simulink model "OFDM_Rx"  (R2025b)
settings: Solver=FixedStepAuto  StartTime=0.0  StopTime=10  RelTol=1e-3
undefined symbols (not defined in the file): Fs, ip, usb
libraries: commofdm x5, hdlsllib x4, plutoradiolib x2, commseqgen3 x2, commchan3 x1, commutil2 x1, commdigbbndpm3 x1, commrandsrc3 x1
settings Model: Creator=joann  LastModifiedBy=joann
settings OptimizationCC: OptimizeBlockIOStorage=off  OptimizeDataStoreBuffers=off  BusAssignmentInplaceUpdate=off
settings DebuggingCC: SFUnexpectedBacktrackingDiag=warning  SFNoUnconditionalDefaultTransitionDiag=warning
settings RTWCC: GenerateReport=on  BuildConfiguration=Debug  LaunchReport=on
settings CodeAppCC: ForceParamTrailComments=on  MATLABSourceComments=on  EnableCustomComments=on
settings GRTTargetCC: MultiInstanceErrorCode=Warning  CombineSignalStateStructs=on  SupportVariableSizeSignals=on

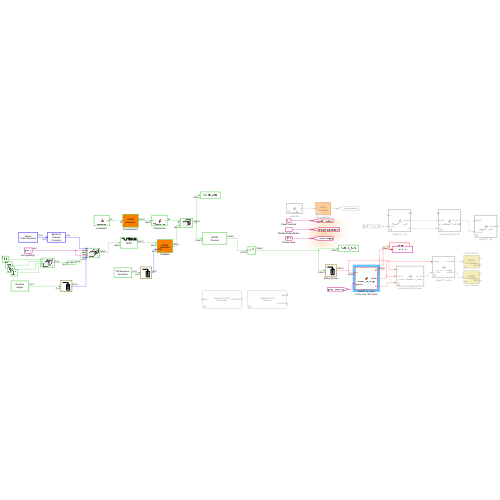
[thumbnail: Simulink's stored preview of the top-level diagram]
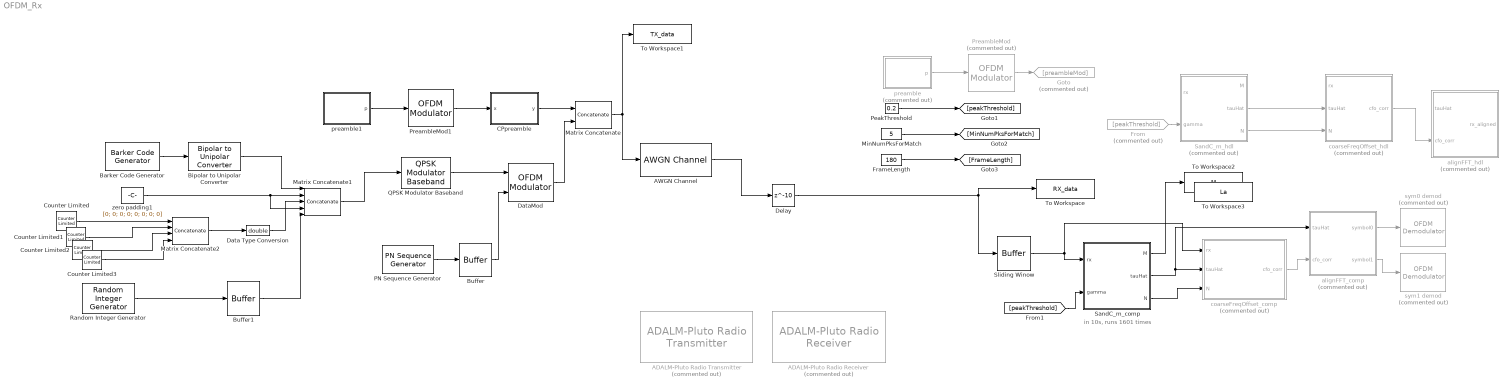
== system OFDM_Rx ==
  note: in 10s, runs 1601 times
  ADALM-Pluto Radio Receiver : plutoradiolib/ADALM-Pluto Radio Receiver  Commented=on  RadioID=usb:0  uri=ip:10.0.0.200  CenterFrequencySource=Dialog  CenterFrequency=868e6  GainSource=AGC Slow Attack  GainSourceBlock=AGC Slow Attack  Gain=10  ChannelMapping=1  BasebandSampleRate=100e3  OutputDataType=double  SamplesPerFrame=160*2*4  OverflowOutputPort=on  EnableBurstMode=off  NumFramesInBurst=2  ShowAdvancedProperties=off  UseCustomFilter=off  filtPathRates=[737280000 11520000 3840000 1920000 960000 240000]  filtCoefficients=[-192 82 85 -215 228 -102 -110 290 -318 145 160 -426 471 -215 -238 633 -697 318 349 -923 1009 -457 -498 1309 -1423 640 693 -1812 1959 -876 -945 2458 -2647 1180 1268 -3290 3534 -1572 -1688 4375 -4698 2091 2247 -5836 6284 -2807 -3031 7918 -8588 3870 4225 -11182 12324 -5662 -6330 17255 -19735 9507 11312 -33568 43355 -25227 -42139 305542 305542 -42139 -25227 43355 -33568 11312 9507 -19735 17255 -6330 -5662 12324 -11182 4225 3870 -8588 7918 -3031 -2807 6284 -5836 2247 2091 -4698 4375 -1688 -1572 3534 -3290 1268 1180 -2647 2458 -945 -876 1959 -1812 693 640 -1423 1309 -498 -457 1009 -923 349 318 -697 633 -238 -215 471 -426 160 145 -318 290 -110 -102 228 -215 85 82 -192]  filtCoefficientSize=128  filtDecimInterpFactor=4  filtGain=-12  filtRFBandwidth=18000000  filterConfigStruct=struct()  EnableQuadratureCorrection=on  EnableRFDCCorrection=on  EnableBasebandDCCorrection=on  FrequencyCorrection=0  OverrideSampleTime=off  SampleTime=0.02  DataTimeout=Inf  ENSMPinControlMode=None  BISTLoopbackMode=Disabled  BISTToneInject=Disabled  BISTSignalGen=PRBS  BISTToneFreq=Fs/32  BISTToneLevel=0
  ADALM-Pluto Radio Transmitter : plutoradiolib/ADALM-Pluto Radio Transmitter  Commented=on  RadioID=usb:0  uri=ip:10.0.0.200  CenterFrequencySource=Dialog  CenterFrequency=868e6  GainSource=Dialog  Gain=-10  ChannelMapping=1  BasebandSampleRate=100e3  UnderflowOutputPort=on  ShowAdvancedProperties=off  UseCustomFilter=off  filtPathRates=[737280000 11520000 3840000 1920000 960000 240000]  filtCoefficients=[-192 82 85 -215 228 -102 -110 290 -318 145 160 -426 471 -215 -238 633 -697 318 349 -923 1009 -457 -498 1309 -1423 640 693 -1812 1959 -876 -945 2458 -2647 1180 1268 -3290 3534 -1572 -1688 4375 -4698 2091 2247 -5836 6284 -2807 -3031 7918 -8588 3870 4225 -11182 12324 -5662 -6330 17255 -19735 9507 11312 -33568 43355 -25227 -42139 305542 305542 -42139 -25227 43355 -33568 11312 9507 -19735 17255 -6330 -5662 12324 -11182 4225 3870 -8588 7918 -3031 -2807 6284 -5836 2247 2091 -4698 4375 -1688 -1572 3534 -3290 1268 1180 -2647 2458 -945 -876 1959 -1812 693 640 -1423 1309 -498 -457 1009 -923 349 318 -697 633 -238 -215 471 -426 160 145 -318 290 -110 -102 228 -215 85 82 -192]  filtCoefficientSize=128  filtDecimInterpFactor=4  filtGain=-12  filtRFBandwidth=18000000  filterConfigStruct=struct()  DataSourceSelect=Input Port  DDSTone1Freq=5e3  DDSTone2Freq=10e3  DDSTone1Scale=0.5  DDSTone2Scale=0.25  DataTimeout=Inf  FrequencyCorrection=0  ENSMPinControlMode=None  BISTLoopbackMode=Disabled  BISTToneInject=Disabled  BISTSignalGen=PRBS  BISTToneFreq=Fs/32  BISTToneLevel=0
  AWGN Channel : commchan3/AWGN Channel  LegacyMode=off  NoiseMethod="Signal to noise ratio  (SNR)"  noiseMode="Signal to noise ratio  (SNR)"  EbNo=10  EsNo=10  SNR=10  BitsPerSymbol=1  SignalPower=1  SpecifySymbolPeriod=off  SamplesPerSymbol=1  SymbolPeriod=1  VarianceSource=Parameter  Variance=1  RandomStream=Global stream  Seed=67  SimulateUsing=Code generation
  Barker Code Generator : commseqgen3/Barker Code Generator  Length=7  LengthSimulink=7  SampleTime=1  SamplesPerFrame=7  OutputDataType=double  SimulateUsing=Code generation
  Bipolar to Unipolar Converter : commutil2/Bipolar to Unipolar Converter  M=2  polarity=Positive  dataType=Inherit via internal rule
  Buffer : Buffer  N=4  OutputFrames=off
  Buffer1 : Buffer  N=21  OutputFrames=off
  CPpreamble : MATLAB Function  TreatAsAtomicUnit=on
  Counter Limited{,1..3} (4 alike) : hdlsllib/Sources/Counter Limited  uplimit=3  tsamp=-1
  Data Type Conversion : DataTypeConversion  OutDataTypeStr=double  SaturateOnIntegerOverflow=off  RndMeth=Floor
  DataMod : commofdm/OFDM Modulator  StatePerturbationForJacobian=1.0e-05  FFTLength=64  NumGuardBandCarriers=[6; 5]  InsertDCNull=on  PilotInputPort=on  PilotCarrierIndices=[12; 26; 40; 54]  CyclicPrefixLength=16  Windowing=on  WindowLength=4  OversamplingFactor=1  NumSymbols=1  NumTransmitAntennas=1  SimulateUsing=Interpreted execution
  Delay : Delay  DelayLength=10  InitialCondition=0
  FrameLength : Constant  Value=180  OutDataTypeStr=int16
  From : From  Commented=on  GotoTag=peakThreshold
  Goto : Goto  Commented=on  GotoTag=preambleMod
  Matrix Concatenate : Concatenate  Mode=Multidimensional array
  Matrix Concatenate1 : Concatenate  NumInputs=5  Mode=Multidimensional array
  Matrix Concatenate2 : Concatenate  NumInputs=4  Mode=Multidimensional array
  MinNumPksForMatch : Constant  Value=5  OutDataTypeStr=int16
  PN Sequence Generator : commseqgen3/PN Sequence Generator  poly='z^8 + z + 1'  ini_sta=[1 0 0 0 1 0 0 1]  outBitMaskSource=Dialog parameter  shift=0  outVarSiz=off  maxOutSizeMode=Dialog parameter  maxOutSize=[10 1]  Ts=1  sampPerFrame=1  reset=off  bitPackedOutputs=off  outDataType=double  numPackedBits=8  bitPackDataSigned=off  bitPackedOutDType=double
      settings: LibrarySourceBlock=|
      | commhdlsource/PN Sequence
      | Generator
  PeakThreshold : Constant  Value=0.2  OutDataTypeStr=double
  PreambleMod : commofdm/OFDM Modulator  Commented=on  StatePerturbationForJacobian=1.0e-05  FFTLength=64  NumGuardBandCarriers=[6; 5]  InsertDCNull=on  PilotInputPort=off  PilotCarrierIndices=[12; 26; 40; 54]  CyclicPrefixLength=0  Windowing=off  WindowLength=4  OversamplingFactor=1  NumSymbols=1  NumTransmitAntennas=1  SimulateUsing=Interpreted execution
  PreambleMod1 : commofdm/OFDM Modulator  StatePerturbationForJacobian=1.0e-05  FFTLength=64  NumGuardBandCarriers=[6; 5]  InsertDCNull=on  PilotInputPort=off  PilotCarrierIndices=[12; 26; 40; 54]  CyclicPrefixLength=0  Windowing=off  WindowLength=4  OversamplingFactor=1  NumSymbols=1  NumTransmitAntennas=1  SimulateUsing=Code generation
  QPSK Modulator Baseband : commdigbbndpm3/QPSK Modulator Baseband  InType=Integer  Enc=Gray  Ph=pi/4  outDtype=double  outWordLen=16  outUDDataType=sfix(16)  outFracLenMode=Best precision  outFracLen=15  outDataTypeStr=double  outLastDataTypeStr=double
      settings: LibrarySourceBlock=|
      | commhdldigbbndpm/QPSK
      | Modulator
      | Baseband
  Random Integer Generator : commrandsrc3/Random Integer Generator  SetSize=4  SeedSource=Auto  Seed=0  SampleTime=1  SamplesPerFrame=1  OutputDataType=double  SimulateUsing=Interpreted execution
  SandC_m_comp : MATLAB Function  TreatAsAtomicUnit=on
  SandC_m_hdl : MATLAB Function  Commented=on  TreatAsAtomicUnit=on
  Sliding Winow : Buffer  N=256  V=255  OutputFrames=off
  To Workspace : ToWorkspace  VariableName=RX_data  SaveFormat=Timeseries  SampleTime=-1
  To Workspace1 : ToWorkspace  VariableName=TX_data  SaveFormat=Timeseries  SampleTime=-1
  To Workspace2 : ToWorkspace  VariableName=M  SaveFormat=Timeseries  SampleTime=-1
  To Workspace3 : ToWorkspace  VariableName=La  SaveFormat=Timeseries  SampleTime=-1
  alignFFT_comp : MATLAB Function  Commented=on  TreatAsAtomicUnit=on
  alignFFT_hdl : MATLAB Function  Commented=on  TreatAsAtomicUnit=on
  coarseFreqOffset_comp : MATLAB Function  Commented=on  TreatAsAtomicUnit=on
  coarseFreqOffset_hdl : MATLAB Function  Commented=on  TreatAsAtomicUnit=on
  preamble : MATLAB Function  Commented=on  TreatAsAtomicUnit=on
  preamble1 : MATLAB Function  TreatAsAtomicUnit=on
  sym0 demod : commofdm/OFDM Demodulator  Commented=on  StatePerturbationForJacobian=1.0e-05  FFTLength=64  NumGuardBandCarriers=[6; 5]  RemoveDCCarrier=off  PilotOutputPort=on  PilotCarrierIndices=[12; 26; 40; 54]  CyclicPrefixLength=16  OversamplingFactor=1  NumSymbols=1  NumReceiveAntennas=1  SimulateUsing=Interpreted execution
  sym1 demod : commofdm/OFDM Demodulator  Commented=on  StatePerturbationForJacobian=1.0e-05  FFTLength=64  NumGuardBandCarriers=[6; 5]  RemoveDCCarrier=off  PilotOutputPort=on  PilotCarrierIndices=[12; 26; 40; 54]  CyclicPrefixLength=16  OversamplingFactor=1  NumSymbols=1  NumReceiveAntennas=1  SimulateUsing=Interpreted execution
  zero padding1 : Constant  Value=[0; 0; 0; 0; 0; 0; 0; 0]  VectorParams1D=off
  wires:
  Delay/1 -> Sliding Winow/1, To Workspace/1
  FrameLength/1 -> [FrameLength]
  PeakThreshold/1 -> [peakThreshold]
  MinNumPksForMatch/1 -> [MinNumPksForMatch]
  Sliding Winow/1 -> SandC_m_comp/1(rx), coarseFreqOffset_comp/1(rx)
  From/1 -> SandC_m_hdl/2(gamma)
  preamble/1(p) -> PreambleMod/1
  PreambleMod/1 -> Goto/1
  SandC_m_hdl/2(tauHat) -> coarseFreqOffset_hdl/2(tauHat)
  SandC_m_hdl/3(N) -> coarseFreqOffset_hdl/3(N)
  coarseFreqOffset_hdl/1(cfo_corr) -> alignFFT_hdl/2(cfo_corr)
  [peakThreshold] -> SandC_m_comp/2(gamma)
  SandC_m_comp/3(N) -> coarseFreqOffset_comp/3(N)
  coarseFreqOffset_comp/1(cfo_corr) -> alignFFT_comp/2(cfo_corr)
  alignFFT_comp/1(symbol0) -> sym0 demod/1
  alignFFT_comp/2(symbol1) -> sym1 demod/1
  SandC_m_comp/2(tauHat) -> alignFFT_comp/1(tauHat), coarseFreqOffset_comp/2(tauHat)
  Counter Limited/1 -> Matrix Concatenate2/1
  Matrix Concatenate2/1 -> Data Type Conversion/1
  Bipolar to Unipolar Converter/1 -> Matrix Concatenate1/1
  DataMod/1 -> Matrix Concatenate/2
  QPSK Modulator Baseband/1 -> DataMod/1
  Matrix Concatenate1/1 -> QPSK Modulator Baseband/1
  Data Type Conversion/1 -> Matrix Concatenate1/3
  Buffer1/1 -> Matrix Concatenate1/5
  preamble1/1(p) -> PreambleMod1/1
  Matrix Concatenate/1 -> AWGN Channel/1, To Workspace1/1
  PreambleMod1/1 -> CPpreamble/1(x)
  CPpreamble/1(y) -> Matrix Concatenate/1
  Counter Limited3/1 -> Matrix Concatenate2/4
  Barker Code Generator/1 -> Bipolar to Unipolar Converter/1
  PN Sequence Generator/1 -> Buffer/1
  Buffer/1 -> DataMod/2
  Counter Limited2/1 -> Matrix Concatenate2/3
  Counter Limited1/1 -> Matrix Concatenate2/2
  zero padding1/1 -> Matrix Concatenate1/4, Matrix Concatenate1/2
  Random Integer Generator/1 -> Buffer1/1
  SandC_m_comp/1(M) -> To Workspace2/1
  AWGN Channel/1 -> Delay/1
  ? -> To Workspace3/1

== matlab function OFDM_Rx/coarseFreqOffset_hdl ==
  data: rx input; tauHat input; N input; cfo_corr output
function cfo_corr  = coarseFreqOffset_hdl(rx, tauHat, N)
%#codegen

% https://dspillustrations.com/pages/posts/misc/schmidlcox-synchronization-for-ofdm.html
% Microsoft Copilot
% https://www.mathworks.com/help/releases/R2025b/comm/ref/pskmod.html

% tunable variables
%half = 32; % each preamble half is 32 units long
%oversample = 4; % oversampling factor
%N = half*oversample; % repeated values

L = length(rx);

if tauHat >= 0 && (tauHat + 2*N) <= L
    
    % repeated halves locations
    h1 = rx(tauHat + (1:N));
    h2 = rx(tauHat + N + (1:N));

    % determine phase angle
    phaseAngle = angle(sum(conj(rx(1: N)) .* rx(N+(1:N))));
    
    % estimated freq offset
    e_hat = phaseAngle/(2*pi*N);
    
    % correct rotation
    n = (0:L-1).';
    cfo_corr = rx .* exp(-1j*2*pi*e_hat*n);
else
    cfo_corr = rx;
end

end

== matlab function OFDM_Rx/SandC_m_hdl ==
  data: M output; rx input; tauHat output; N output; gamma input
function [M,tauHat, N] = SandC_m_hdl(rx, gamma)
%#codegen

half = 32; % each preamble half is 32 units long
oversample = 4; % oversampling factor
N = half*oversample; % repeated values

rx = rx(:);
L = length(rx); 
La = L - 2*N;

% handling a case of 0 or negative numbers if buffer does something weird
if La < 1
    tauHat = -1;
    M = 0;
    return;
end

% cross correlate
P = complex(zeros(La + 1,1));
R = zeros(La + 1,1);
M = (zeros(La + 1,1));
%MPeak = complex(1);

for d = 1 : (La +1)
    r1 = rx(d : d+N-1);
    r2 = rx(d+N : d+2*N-1);

    P(d) = sum(conj(r1).*r2);
    R(d) = sum(abs(r2).^2);
    M(d) = abs(P(d))^2 / (R(d)^2 + 1e-12); % 1e-12 used to keep from num/0
end

% finding timing index for FFT alignment
[Mmax, i] = max(M);

if Mmax > gamma
    tauHat = i -1; % -1 to change from 1-based counting to 0-based counting
else
    tauHat = -1;
end
end

== matlab function OFDM_Rx/alignFFT_hdl ==
  data: tauHat input; cfo_corr input; rx_aligned output
function rx_aligned = alignFFT_hdl(tauHat, cfo_corr)
%#codegen

% https://dspillustrations.com/pages/posts/misc/schmidlcox-synchronization-for-ofdm.html
% Microsoft Copilot
% https://www.mathworks.com/help/releases/R2025b/comm/ref/pskmod.html

% Edge cases for tauHat
if isnan(tauHat)
    tauHat = 1;
elseif tauHat > L
    tauHat = mod(tauHat, L);  % Wrap around if tauHat exceeds signal length
end

% Perform the alignment 
rx_aligned = circshift(cfo_corr, -tauHat);  % Shift signal to align the symbol
    
end

== matlab function OFDM_Rx/preamble ==
  data: p output
function p = preamble()
%#codegen

% https://dspillustrations.com/pages/posts/misc/schmidlcox-synchronization-for-ofdm.html
% Microsoft Copilot
% https://www.mathworks.com/help/releases/R2025b/comm/ref/pskmod.html


%p = complex( ...
    %[1; 1; -1; -1; 1; -1; -1; 1; 1; -1; 1; 1; -1; 1; 1;...
    %-1; 1; -1; 1; -1; 1; -1; 1; 1; -1; -1; 0;...
    %1; 1; -1; -1; 1; -1; -1; 1; 1; -1; 1; 1; -1; 1; 1;...
    %-1; 1; -1; 1; -1; 1; -1; 1; 1; -1; -1],0);


L = 64; % FFT Length: 64
M = 4; % Modulation Order
numDataSubc = 53; 

% training symbol (used once to get the raw data symbols)
%randomQAM = qammod(randi([0 1], numDataSubc,1),M,true);
%ramdomQAM(2:2:end) = [0];

randomQAM = [-1.0000e+000 +  1.0000e+000i;
     0.0000e+000 +  0.0000e+000i;
    -1.0000e+000 +  1.0000e+000i;
     0.0000e+000 +  0.0000e+000i;
    -1.0000e+000 -  1.0000e+000i;
     0.0000e+000 +  0.0000e+000i;
    -1.0000e+000 +  1.0000e+000i;
     0.0000e+000 +  0.0000e+000i;
    -1.0000e+000 +  1.0000e+000i;
     0.0000e+000 +  0.0000e+000i;
    -1.0000e+000 -  1.0000e+000i;
     0.0000e+000 +  0.0000e+000i;
    -1.0000e+000 -  1.0000e+000i;
     0.0000e+000 +  0.0000e+000i;
    -1.0000e+000 -  1.0000e+000i;
     0.0000e+000 +  0.0000e+000i;
    -1.0000e+000 -  1.0000e+000i;
     0.0000e+000 +  0.0000e+000i;
    -1.0000e+000 +  1.0000e+000i;
     0.0000e+000 +  0.0000e+000i;
    -1.0000e+000 -  1.0000e+000i;
     0.0000e+000 +  0.0000e+000i;
    -1.0000e+000 +  1.0000e+000i;
     0.0000e+000 +  0.0000e+000i;
    -1.0000e+000 +  1.0000e+000i;
     0.0000e+000 +  0.0000e+000i;
    -1.0000e+000 -  1.0000e+000i;
     0.0000e+000 +  0.0000e+000i;
    -1.0000e+000 +  1.0000e+000i;
     0.0000e+000 +  0.0000e+000i;
    -1.0000e+000 -  1.0000e+000i;
     0.0000e+000 +  0.0000e+000i;
    -1.0000e+000 -  1.0000e+000i;
     0.0000e+000 +  0.0000e+000i;
    -1.0000e+000 +  1.0000e+000i;
     0.0000e+000 +  0.0000e+000i;
    -1.0000e+000 -  1.0000e+000i;
     0.0000e+000 +  0.0000e+000i;
    -1.0000e+000 -  1.0000e+000i;
     0.0000e+000 +  0.0000e+000i;
    -1.0000e+000 -  1.0000e+000i;
     0.0000e+000 +  0.0000e+000i;
    -1.0000e+000 -  1.0000e+000i;
     0.0000e+000 +  0.0000e+000i;
    -1.0000e+000 +  1.0000e+000i;
     0.0000e+000 +  0.0000e+000i;
    -1.0000e+000 +  1.0000e+000i;
     0.0000e+000 +  0.0000e+000i;
    -1.0000e+000 -  1.0000e+000i;
     0.0000e+000 +  0.0000e+000i;
    -1.0000e+000 -  1.0000e+000i;
     0.0000e+000 +  0.0000e+000i]; 

p = sqrt(2)*randomQAM;
end

== matlab function OFDM_Rx/SandC_m_comp ==
  data: rx input; M output; gamma input; tauHat output; N output
function [M, tauHat, N] = SandC_m_comp(rx, gamma)

half = 32; % each preamble half is 32 units long
oversample = 4; % oversampling factor
N = half*oversample; % repeated values = 32*4 = 128

rx = rx(:); % 256
L = length(rx); 
La = L - 2*N;

% holding tauHat value for valid frame detection
persistent tauHat_prev
if isempty(tauHat_prev)
    tauHat_prev = 1;
end

% handling a case of 0 or negative numbers if buffer does something weird
if La < 1
    tauHat = tauHat_prev;
    M = 0;
    return;
end

% cross correlate
P = complex(zeros(La + 1,1));
R = zeros(La + 1,1);
M = zeros(La + 1,1);
%MPeak = complex(1);

for d = 1 : (La +1)
    r1 = rx(d : d+N-1);
    r2 = rx(d+N : d+2*N-1);

    P(d) = sum(conj(r1).*r2);
    R(d) = sum(abs(r2).^2);
    M(d) = abs(P(d))^2 / (R(d)^2 + 1e-12); % 1e-12 used to keep from num/0
end

% finding timing index for FFT alignment
[Mmax, i] = max(M);

if Mmax > gamma
    tauHat = i -1; % -1 to change from 1-based counting to 0-based counting
    tauHat_prev = tauHat;
else
    tauHat = tauHat_prev; % new tauHat is previous valid tauHat
end

end

== matlab function OFDM_Rx/coarseFreqOffset_comp ==
  data: rx input; cfo_corr output; tauHat input; N input
function cfo_corr  = coarseFreqOffset_comp(rx, tauHat, N)

% https://dspillustrations.com/pages/posts/misc/schmidlcox-synchronization-for-ofdm.html
% Microsoft Copilot
% https://www.mathworks.com/help/releases/R2025b/comm/ref/pskmod.html

% tunable variables
%half = 32; % each preamble half is 32 units long
%oversample = 4; % oversampling factor
%N = half*oversample; % repeated values

L = length(rx);

if tauHat >= 0 && (tauHat + 2*N) <= L
    
    % repeated halves locations
    h1 = rx(tauHat + (1:N));
    h2 = rx(tauHat + N + (1:N));

    % determine phase angle
    phaseAngle = angle(sum(conj(h1) .* h2));
    
    % estimated freq offset
    e_hat = phaseAngle/(2*pi*N);
    
    % correct rotation
    n = (0:L-1).';
    cfo_corr = rx .* exp(-1j*2*pi*e_hat*n);
else
    cfo_corr = rx;
end

end

== matlab function OFDM_Rx/alignFFT_comp ==
  data: tauHat input; symbol0 output; cfo_corr input; symbol1 output
function [symbol0, symbol1] = alignFFT_comp(tauHat, cfo_corr)
%#codegen

% https://dspillustrations.com/pages/posts/misc/schmidlcox-synchronization-for-ofdm.html
% Microsoft Copilot
% https://www.mathworks.com/help/releases/R2025b/comm/ref/pskmod.html

% tunable variables
oversample = 4;
CPLen = 16; % cyclic prefix length w/o oversampling
Nfft = 64; % FFT size before oversampling

% OFDM and sampling calculations
CPLen_os = CPLen * oversample; % 64 -> oversampled cyclic prefix length
Nfft_os = Nfft *oversample; % 64*4 = 256 samples total
symbol_os = (Nfft + CPLen) *oversample; % (64+16)*4 = 320 samples total

tauHat = tauHat + (Nfft_os/2); % centering tauHat in preamble plateau

if tauHat >= 0
    % starting of OFDM symbols (including CP)
    symbol_0_CPstart = (tauHat +1) - CPLen_os;
    symbol_0_FFTstart = symbol_0_CPstart + CPLen_os; 
    symbol_1_CPstart = symbol_0_CPstart + symbol_os;
    symbol_1_FFTstart = symbol_1_CPstart + CPLen_os;
    
    % actual symbols
    symbol_0_os = cfo_corr(symbol_0_CPstart+1 : symbol_0_CPstart +symbol_os);
    symbol_1_os = cfo_corr(symbol_1_CPstart+1 : symbol_1_CPstart +symbol_os);
    % symbol_0_os = cfo_corr(symbol_0_FFTstart+1 : symbol_0_FFTstart +Nfft_os);
    % symbol_1_os = cfo_corr(symbol_1_FFTstart+1 : symbol_1_FFTstart +Nfft_os);
    
    symbol0 = symbol_0_os(1:oversample:end);
    symbol1 = symbol_1_os(1:oversample:end);
% else
%     return;
end

end

== matlab function OFDM_Rx/CPpreamble ==
  data: y output; x input
function y = CPpreamble(x)
%#codegen

Nfft = 64; % FFT Length (also # of subcarriers)
CP = 16; % Cyclic Prefix Length

half = x(1:Nfft/2);
preambleNoCP = [half;half];
y = [preambleNoCP(end-CP+1:end);preambleNoCP];
end

== matlab function OFDM_Rx/preamble1 ==
  data: p output
function p = preamble()
%#codegen

% https://dspillustrations.com/pages/posts/misc/schmidlcox-synchronization-for-ofdm.html
% Microsoft Copilot
% https://www.mathworks.com/help/releases/R2025b/comm/ref/pskmod.html


%p = complex( ...
    %[1; 1; -1; -1; 1; -1; -1; 1; 1; -1; 1; 1; -1; 1; 1;...
    %-1; 1; -1; 1; -1; 1; -1; 1; 1; -1; -1; 0;...
    %1; 1; -1; -1; 1; -1; -1; 1; 1; -1; 1; 1; -1; 1; 1;...
    %-1; 1; -1; 1; -1; 1; -1; 1; 1; -1; -1],0);


L = 64; % FFT Length: 64
M = 4; % Modulation Order
numDataSubc = 53; 

% training symbol (used once to get the raw data symbols)
%randomQAM = qammod(randi([0 1], numDataSubc,1),M,true);
%ramdomQAM(2:2:end) = [0];

randomQAM = [-1.0000e+000 +  1.0000e+000i;
     0.0000e+000 +  0.0000e+000i;
    -1.0000e+000 +  1.0000e+000i;
     0.0000e+000 +  0.0000e+000i;
    -1.0000e+000 -  1.0000e+000i;
     0.0000e+000 +  0.0000e+000i;
    -1.0000e+000 +  1.0000e+000i;
     0.0000e+000 +  0.0000e+000i;
    -1.0000e+000 +  1.0000e+000i;
     0.0000e+000 +  0.0000e+000i;
    -1.0000e+000 -  1.0000e+000i;
     0.0000e+000 +  0.0000e+000i;
    -1.0000e+000 -  1.0000e+000i;
     0.0000e+000 +  0.0000e+000i;
    -1.0000e+000 -  1.0000e+000i;
     0.0000e+000 +  0.0000e+000i;
    -1.0000e+000 -  1.0000e+000i;
     0.0000e+000 +  0.0000e+000i;
    -1.0000e+000 +  1.0000e+000i;
     0.0000e+000 +  0.0000e+000i;
    -1.0000e+000 -  1.0000e+000i;
     0.0000e+000 +  0.0000e+000i;
    -1.0000e+000 +  1.0000e+000i;
     0.0000e+000 +  0.0000e+000i;
    -1.0000e+000 +  1.0000e+000i;
     0.0000e+000 +  0.0000e+000i;
    -1.0000e+000 -  1.0000e+000i;
     0.0000e+000 +  0.0000e+000i;
    -1.0000e+000 +  1.0000e+000i;
     0.0000e+000 +  0.0000e+000i;
    -1.0000e+000 -  1.0000e+000i;
     0.0000e+000 +  0.0000e+000i;
    -1.0000e+000 -  1.0000e+000i;
     0.0000e+000 +  0.0000e+000i;
    -1.0000e+000 +  1.0000e+000i;
     0.0000e+000 +  0.0000e+000i;
    -1.0000e+000 -  1.0000e+000i;
     0.0000e+000 +  0.0000e+000i;
    -1.0000e+000 -  1.0000e+000i;
     0.0000e+000 +  0.0000e+000i;
    -1.0000e+000 -  1.0000e+000i;
     0.0000e+000 +  0.0000e+000i;
    -1.0000e+000 -  1.0000e+000i;
     0.0000e+000 +  0.0000e+000i;
    -1.0000e+000 +  1.0000e+000i;
     0.0000e+000 +  0.0000e+000i;
    -1.0000e+000 +  1.0000e+000i;
     0.0000e+000 +  0.0000e+000i;
    -1.0000e+000 -  1.0000e+000i;
     0.0000e+000 +  0.0000e+000i;
    -1.0000e+000 -  1.0000e+000i;
     0.0000e+000 +  0.0000e+000i]; 

p = sqrt(2)*randomQAM;
end
